simulink model "control_input"  (R2015a)
settings: Solver=ode45  StartTime=0.0  StopTime=10.0  RelTol=1e-3
values from neighbouring files (symbols this model uses):
  Ec = Ec / Ec    [control_input_main.m]
  Kc = Kc*0    [control_input_main.m]
undefined symbols (not defined in the file or in its folder): A, B, C
settings Model: Creator=Elca  LastModifiedBy=Elca

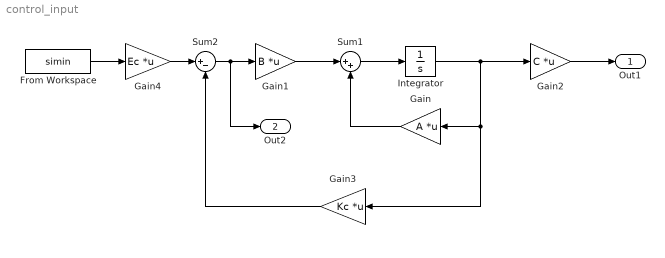
== system control_input ==
  From Workspace : FromWorkspace  VariableName=simin  SampleTime=0
  Gain : Gain  Gain=A  Multiplication=Matrix(K*u)
  Gain1 : Gain  Gain=B  Multiplication=Matrix(K*u)
  Gain2 : Gain  Gain=C  Multiplication=Matrix(K*u)
  Gain3 : Gain  Gain=Kc  Multiplication=Matrix(K*u)
  Gain4 : Gain  Gain=Ec  Multiplication=Matrix(K*u)
  Integrator : Integrator
  Sum1 : Sum  Inputs=|++
  Sum2 : Sum  Inputs=|+-
  Out1 : Outport
  Out2 : Outport  Port=2
  wires:
  Integrator/1 -> Gain3/1, Gain/1, Gain2/1
  Gain1/1 -> Sum1/1
  Sum1/1 -> Integrator/1
  Gain/1 -> Sum1/2
  Gain2/1 -> Out1/1
  From Workspace/1 -> Gain4/1
  Sum2/1 -> Out2/1, Gain1/1
  Gain4/1 -> Sum2/1
  Gain3/1 -> Sum2/2
